simulink subsystem "c50In"  (R2023b)
settings: Solver=VariableStepAuto  StartTime=0.0  StopTime=10.0  RelTol=1e-3
libraries: Raptor_lib x5
settings Model: Creator=serga  LastModifiedBy=serga

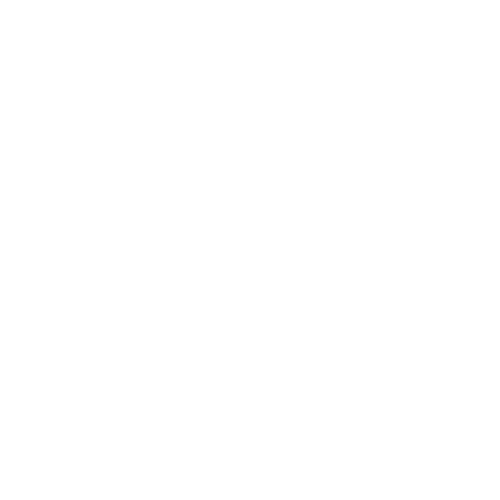
[thumbnail: Simulink's stored preview of the top-level diagram]
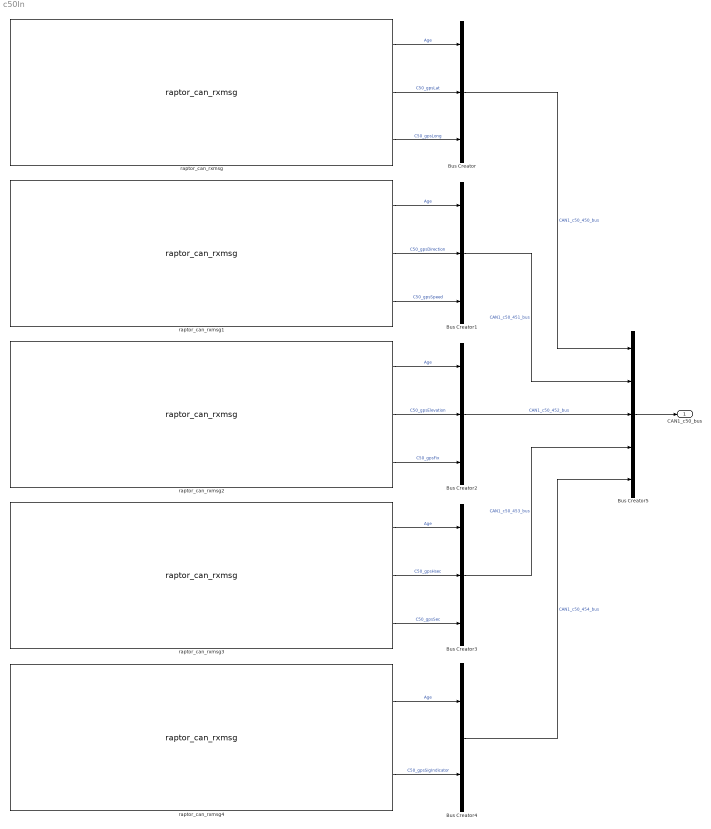
== system c50In ==
  Bus Creator{,1..3} (4 alike) : BusCreator  Inputs=3
  Bus Creator4 : BusCreator  Inputs=2
  Bus Creator5 : BusCreator  Inputs=5
  raptor_can_rxmsg : Raptor_lib/CAN/raptor_can_rxmsg  canDefinition=struct('dbcFile', 'raptor_CAN1.dbc','message', 'C50_450','comment', '','signals', {{'C50_gpsLat','C50_gpsLong'}},'enabled', [ 1 1;],'scaled', [ 1 1;],'canBus', '''CAN1''','messageID', [ 450;],'idMask', [ 536870911;],'payloadMask', [],'payloadValue', [],'period', [ 0;],'mailbox', '''''','queueSize', [ 1;],'label', [ 1;],'ver', [ 2;],'showID', [ 0;],'showRaw', [ 0;],'showRawMsg', [ 0;],'useStartVals', [ 0;],'extendedId', [ 0;],'showAge', [ 1;],'useSimFunc', [ 0;],'sim_func_name', '''''','fill', [ 0;],'editID', [ 0;],'signalOrder', [ 1;],'signalAscDes', [ 1;],'msgLength', [ 8;])  canBus='CAN1'  mailbox=''  payloadMask=[]  payloadValue=[]  idMask=hex2dec('1FFFFFFF')  queueSize=1  showID=0  label=1  fill=0  id=450  showRaw=0  showAge=1  signalOrder=1  signalInfo={{struct('Name', 'C50_gpsLong','StartBit', [ 32;],'SignalSize', [ 32;],'ByteOrder', 'LittleEndian','ValueType', 'SIGNED','Class', 'int32','Signed', [ 1;],'Factor', [ 1;],'Offset', [ 0;],'Min', [ -180;],'Max', [ 180;],'Units', 'NDEG','StartVal', [ 0;],'Comment', 'Longitude in NDEG: +/-[degree][min].[sec/60]','Multiplexed', [ 0;],'Multiplexor', [ 0;],'MultiplexMode_Min', [ 0;],'MultiplexMode_Max', [ 0;]),struct('Name', 'C50_gpsLat','StartBit', [ 0;],'SignalSize', [ 32;],'ByteOrder', 'LittleEndian','ValueType', 'SIGNED','Class', 'int32','Signed', [ 1;],'Factor', [ 1;],'Offset', [ 0;],'Min', [ -90;],'Max', [ 90;],'Units', 'NDEG','StartVal', [ 0;],'Comment', 'Latitude in NDEG: +/-[degree][min].[sec/60]','Multiplexed', [ 0;],'Multiplexor', [ 0;],'MultiplexMode_Min', [ 0;],'MultiplexMode_Max', [ 0;])}}  showRawMsg=0  useSimFunc=0  sim_func_name=''  useStartVals=0  extendedId=0
      settings: SourceProductName=Raptor
  raptor_can_rxmsg1 : Raptor_lib/CAN/raptor_can_rxmsg  canDefinition=struct('dbcFile', 'raptor_CAN1.dbc','message', 'C50_451','comment', '','signals', {{'C50_gpsDirection','C50_gpsSpeed'}},'enabled', [ 1 1;],'scaled', [ 1 1;],'canBus', '''CAN1''','messageID', [ 451;],'idMask', [ 536870911;],'payloadMask', [],'payloadValue', [],'period', [ 0;],'mailbox', '''''','queueSize', [ 1;],'label', [ 1;],'ver', [ 2;],'showID', [ 0;],'showRaw', [ 0;],'showRawMsg', [ 0;],'useStartVals', [ 0;],'extendedId', [ 0;],'showAge', [ 1;],'useSimFunc', [ 0;],'sim_func_name', '''''','fill', [ 0;],'editID', [ 0;],'signalOrder', [ 1;],'signalAscDes', [ 1;],'msgLength', [ 8;])  canBus='CAN1'  mailbox=''  payloadMask=[]  payloadValue=[]  idMask=hex2dec('1FFFFFFF')  queueSize=1  showID=0  label=1  fill=0  id=451  showRaw=0  showAge=1  signalOrder=1  signalInfo={{struct('Name', 'C50_gpsDirection','StartBit', [ 32;],'SignalSize', [ 32;],'ByteOrder', 'LittleEndian','ValueType', 'SIGNED','Class', 'int32','Signed', [ 1;],'Factor', [ 1;],'Offset', [ 0;],'Min', [ -360;],'Max', [ 360;],'Units', 'degrees','StartVal', [ 0;],'Comment', 'Track angle in degrees','Multiplexed', [ 0;],'Multiplexor', [ 0;],'MultiplexMode_Min', [ 0;],'MultiplexMode_Max', [ 0;]),struct('Name', 'C50_gpsSpeed','StartBit', [ 0;],'SignalSize', [ 32;],'ByteOrder', 'LittleEndian','ValueType', 'SIGNED','Class', 'int32','Signed', [ 1;],'Factor', [ 1;],'Offset', [ 0;],'Min', [ 0;],'Max', [ 0;],'Units', 'kph','StartVal', [ 0;],'Comment', 'Speed over the ground in kph','Multiplexed', [ 0;],'Multiplexor', [ 0;],'MultiplexMode_Min', [ 0;],'MultiplexMode_Max', [ 0;])}}  showRawMsg=0  useSimFunc=0  sim_func_name=''  useStartVals=0  extendedId=0
      settings: SourceProductName=Raptor
  raptor_can_rxmsg2 : Raptor_lib/CAN/raptor_can_rxmsg  canDefinition=struct('dbcFile', 'raptor_CAN1.dbc','message', 'C50_452','comment', '','signals', {{'C50_gpsElevation','C50_gpsFix'}},'enabled', [ 1 1;],'scaled', [ 1 1;],'canBus', '''CAN1''','messageID', [ 452;],'idMask', [ 536870911;],'payloadMask', [],'payloadValue', [],'period', [ 0;],'mailbox', '''''','queueSize', [ 1;],'label', [ 1;],'ver', [ 2;],'showID', [ 0;],'showRaw', [ 0;],'showRawMsg', [ 0;],'useStartVals', [ 0;],'extendedId', [ 0;],'showAge', [ 1;],'useSimFunc', [ 0;],'sim_func_name', '''''','fill', [ 0;],'editID', [ 0;],'signalOrder', [ 1;],'signalAscDes', [ 1;],'msgLength', [ 8;])  canBus='CAN1'  mailbox=''  payloadMask=[]  payloadValue=[]  idMask=hex2dec('1FFFFFFF')  queueSize=1  showID=0  label=1  fill=0  id=452  showRaw=0  showAge=1  signalOrder=1  signalInfo={{struct('Name', 'C50_gpsElevation','StartBit', [ 0;],'SignalSize', [ 32;],'ByteOrder', 'LittleEndian','ValueType', 'SIGNED','Class', 'int32','Signed', [ 1;],'Factor', [ 1;],'Offset', [ 0;],'Min', [ -5000;],'Max', [ 5000;],'Units', 'm','StartVal', [ 0;],'Comment', 'Antenna altitude above/below mean sea level (geoid) in meters','Multiplexed', [ 0;],'Multiplexor', [ 0;],'MultiplexMode_Min', [ 0;],'MultiplexMode_Max', [ 0;]),struct('Name', 'C50_gpsFix','StartBit', [ 32;],'SignalSize', [ 32;],'ByteOrder', 'LittleEndian','ValueType', 'UNSIGNED','Class', 'uint32','Signed', [ 0;],'Factor', [ 1;],'Offset', [ 0;],'Min', [ 0;],'Max', [ 3;],'Units', '','StartVal', [ 0;],'Comment', 'Operating mode, used for navigation (1 = Fix not available; 2 = 2D; 3 = 3D)','Multiplexed', [ 0;],'Multiplexor', [ 0;],'MultiplexMode_Min', [ 0;],'MultiplexMode_Max', [ 0;])}}  showRawMsg=0  useSimFunc=0  sim_func_name=''  useStartVals=0  extendedId=0
      settings: SourceProductName=Raptor
  raptor_can_rxmsg3 : Raptor_lib/CAN/raptor_can_rxmsg  canDefinition=struct('dbcFile', 'raptor_CAN1.dbc','message', 'C50_453','comment', '','signals', {{'C50_gpsHsec','C50_gpsSec'}},'enabled', [ 1 1;],'scaled', [ 1 1;],'canBus', '''CAN1''','messageID', [ 453;],'idMask', [ 536870911;],'payloadMask', [],'payloadValue', [],'period', [ 0;],'mailbox', '''''','queueSize', [ 1;],'label', [ 1;],'ver', [ 2;],'showID', [ 0;],'showRaw', [ 0;],'showRawMsg', [ 0;],'useStartVals', [ 0;],'extendedId', [ 0;],'showAge', [ 1;],'useSimFunc', [ 0;],'sim_func_name', '''''','fill', [ 0;],'editID', [ 0;],'signalOrder', [ 1;],'signalAscDes', [ 1;],'msgLength', [ 8;])  canBus='CAN1'  mailbox=''  payloadMask=[]  payloadValue=[]  idMask=hex2dec('1FFFFFFF')  queueSize=1  showID=0  label=1  fill=0  id=453  showRaw=0  showAge=1  signalOrder=1  signalInfo={{struct('Name', 'C50_gpsHsec','StartBit', [ 0;],'SignalSize', [ 32;],'ByteOrder', 'LittleEndian','ValueType', 'UNSIGNED','Class', 'uint32','Signed', [ 0;],'Factor', [ 1;],'Offset', [ 0;],'Min', [ 0;],'Max', [ 99;],'Units', 'hsec','StartVal', [ 0;],'Comment', 'Hundredth part of a second','Multiplexed', [ 0;],'Multiplexor', [ 0;],'MultiplexMode_Min', [ 0;],'MultiplexMode_Max', [ 0;]),struct('Name', 'C50_gpsSec','StartBit', [ 32;],'SignalSize', [ 32;],'ByteOrder', 'LittleEndian','ValueType', 'UNSIGNED','Class', 'uint32','Signed', [ 0;],'Factor', [ 1;],'Offset', [ 0;],'Min', [ 0;],'Max', [ 59;],'Units', 'sec','StartVal', [ 0;],'Comment', 'Seconds after the minute','Multiplexed', [ 0;],'Multiplexor', [ 0;],'MultiplexMode_Min', [ 0;],'MultiplexMode_Max', [ 0;])}}  showRawMsg=0  useSimFunc=0  sim_func_name=''  useStartVals=0  extendedId=0
      settings: SourceProductName=Raptor
  raptor_can_rxmsg4 : Raptor_lib/CAN/raptor_can_rxmsg  canDefinition=struct('dbcFile', 'raptor_CAN1.dbc','message', 'C50_454','comment', '','signals', {{'C50_gpsSigIndicator'}},'enabled', [ 1;],'scaled', [ 1;],'canBus', '''CAN1''','messageID', [ 454;],'idMask', [ 536870911;],'payloadMask', [],'payloadValue', [],'period', [ 0;],'mailbox', '''''','queueSize', [ 1;],'label', [ 1;],'ver', [ 2;],'showID', [ 0;],'showRaw', [ 0;],'showRawMsg', [ 0;],'useStartVals', [ 0;],'extendedId', [ 0;],'showAge', [ 1;],'useSimFunc', [ 0;],'sim_func_name', '''''','fill', [ 0;],'editID', [ 0;],'signalOrder', [ 1;],'signalAscDes', [ 1;],'msgLength', [ 8;])  canBus='CAN1'  mailbox=''  payloadMask=[]  payloadValue=[]  idMask=hex2dec('1FFFFFFF')  queueSize=1  showID=0  label=1  fill=0  id=454  showRaw=0  showAge=1  signalOrder=1  signalInfo={{struct('Name', 'C50_gpsSigIndicator','StartBit', [ 0;],'SignalSize', [ 32;],'ByteOrder', 'LittleEndian','ValueType', 'UNSIGNED','Class', 'uint32','Signed', [ 0;],'Factor', [ 1;],'Offset', [ 0;],'Min', [ 0;],'Max', [ 3;],'Units', '','StartVal', [ 0;],'Comment', 'GPS quality indicator (0 = Invalid; 1 = Fix; 2 = Differential; 3 = Sensitive)','Multiplexed', [ 0;],'Multiplexor', [ 0;],'MultiplexMode_Min', [ 0;],'MultiplexMode_Max', [ 0;])}}  showRawMsg=0  useSimFunc=0  sim_func_name=''  useStartVals=0  extendedId=0
      settings: SourceProductName=Raptor
  CAN1_c50_bus : Outport
  wires:
  raptor_can_rxmsg/1 -> Bus Creator/1  "Age"
  raptor_can_rxmsg/2 -> Bus Creator/2  "C50_gpsLat"
  raptor_can_rxmsg/3 -> Bus Creator/3  "C50_gpsLong"
  raptor_can_rxmsg1/1 -> Bus Creator1/1  "Age"
  raptor_can_rxmsg1/2 -> Bus Creator1/2  "C50_gpsDirection"
  raptor_can_rxmsg1/3 -> Bus Creator1/3  "C50_gpsSpeed"
  raptor_can_rxmsg2/1 -> Bus Creator2/1  "Age"
  raptor_can_rxmsg2/2 -> Bus Creator2/2  "C50_gpsElevation"
  raptor_can_rxmsg2/3 -> Bus Creator2/3  "C50_gpsFix"
  raptor_can_rxmsg3/1 -> Bus Creator3/1  "Age"
  raptor_can_rxmsg3/2 -> Bus Creator3/2  "C50_gpsHsec"
  raptor_can_rxmsg3/3 -> Bus Creator3/3  "C50_gpsSec"
  raptor_can_rxmsg4/1 -> Bus Creator4/1  "Age"
  raptor_can_rxmsg4/2 -> Bus Creator4/2  "C50_gpsSigIndicator"
  Bus Creator/1 -> Bus Creator5/1  "CAN1_c50_450_bus"
  Bus Creator1/1 -> Bus Creator5/2  "CAN1_c50_451_bus"
  Bus Creator2/1 -> Bus Creator5/3  "CAN1_c50_452_bus"
  Bus Creator3/1 -> Bus Creator5/4  "CAN1_c50_453_bus"
  Bus Creator4/1 -> Bus Creator5/5  "CAN1_c50_454_bus"
  Bus Creator5/1 -> CAN1_c50_bus/1
